simulink model "DutyRelay"  (Simulink 7.0)
settings: Solver=FixedStepDiscrete  StartTime=0.0  StopTime=inf  FixedStep=0.5  RelTol=1e-3
libraries: SuperLogic x3, simulink x1, RT x1
settings Model: Creator=ugur  LastModifiedBy=xx  SimulationMode=accelerator
settings DataIOCC: LimitDataPoints=off  OutputSaveName=yout_CPID
settings OptimizationCC: InlineInvariantSignals=on
settings DebuggingCC: SaveWithParameterizedLinksMsg=none  SignalResolutionControl=TryResolveAllWithWarning  MultiTaskDSMMsg=warning  MultiTaskCondExecSysMsg=none  StrictBusMsg=None
settings RTWCC: IncludeERTFirstTime=on
settings GRTTargetCC: TargetFcnLib=ansi_tfl_tmw.mat

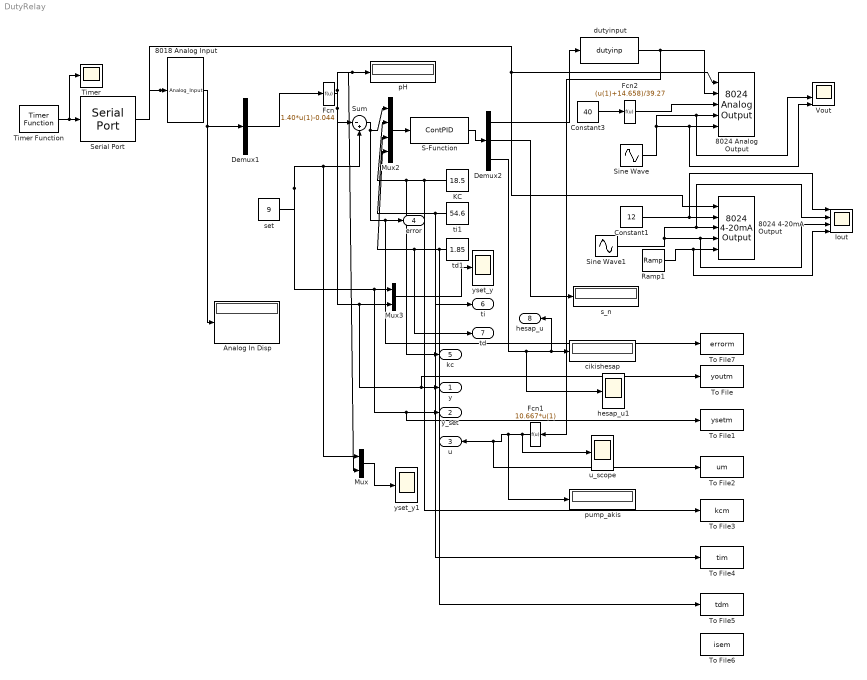
== system DutyRelay ==
  8018 Analog Input : S-Function  FunctionName=Analog_Input  Parameters=AC1, AC2, AC3, AC4, AC5, AC6, AC7, AC8  mask(S function: Analog Input){AC1=off, AC2=on, AC3=off, AC4=off, AC5=off, AC6=off, AC7=off, AC8=off}
      mask prompts: AC1 "Analog Channel 1"; AC2 "Analog Channel 2"; AC3 "Analog Channel 3"; AC4 "Analog Channel 4"; AC5 "Analog Channel 5"; AC6 "Analog Channel 6"; AC7 "Analog Channel 7"; AC8 "Analog Channel 8"
      mask help:
      | This M-file reads the analog input channels from the SL 8018 with 8520
      | The first input is the Com_port number from Serial Port Block.
      mask Display: image(imread('8018.jpg'))
  8024 4-20mA Output : SuperLogic/8024 4-20mA Output  SystemSampleTime=-1  OC1=on  OC2=on  OC3=on  OC4=on
  8024 Analog Output : SuperLogic/8024 Analog Output  SystemSampleTime=-1  OC1=on  OC2=on  OC3=on  OC4=on
  Analog In Disp : Display
  Constant1 : Constant  Value=12  OutDataType=sfix(16)  OutScaling=2^0
  Constant3 : Constant  Value=40  OutDataType=sfix(16)  OutScaling=2^0
  Demux1 : Demux  Outputs=1
  Demux2 : Demux  Outputs=3
  Fcn : Fcn  Expr=1.40*u(1)-0.044
  Fcn1 : Fcn  Orientation=left  Expr=10.667*u(1)
  Fcn2 : Fcn  Expr=(u(1)+14.658)/39.27
  Iout : Scope  NumInputPorts=4
      settings: TimeRange=10  YMin=0~0~0~0  YMax=24~24~24~24  SaveName=ScopeData3  SampleInput=on
  KC : Constant  Orientation=left  Value=18.5  OutDataType=sfix(16)  OutScaling=2^0
  Mux : Mux  Inputs=2
  Mux2 : Mux
  Mux3 : Mux  Inputs=2
  Ramp1 : simulink/Sources/Ramp  SystemSampleTime=-1  slope=0.5  start=0  X0=4
  S-Function : S-Function  FunctionName=ContPID  Parameters=dperiod
  Serial Port : SuperLogic/Serial Port  PORT_NAME=COM1  PORT_BRATE=19200
  Sine Wave : Sin  Amplitude=4  Bias=6  Frequency=pi/5  SampleTime=0
  Sine Wave1 : Sin  Amplitude=8  Bias=12  Frequency=pi/5  SampleTime=0
  Sum : Sum  Inputs=|-+  OutDataType=sfix(16)  OutScaling=2^0
  Timer : Scope
      settings: TimeRange=30  YMin=0  YMax=500
  Timer Function : RT/Timer Function  Priority=245354192  step=500  tmrpriority=HIGH  ThPriority=NORMAL
  To File : ToFile  Filename=youtm
  To File1 : ToFile  Filename=ysetm
  To File2 : ToFile  Filename=um
  To File3 : ToFile  Filename=kcm
  To File4 : ToFile  Filename=tim
  To File5 : ToFile  Filename=tdm
  To File6 : ToFile  Filename=isem
  To File7 : ToFile  Filename=errorm
  Vout : Scope  NumInputPorts=4
      settings: TimeRange=10  YMin=0~0~0~0  YMax=10~10~10~10  SaveName=ScopeData2  SampleInput=on
  cikishesap : Display
  dutyinput : S-Function  FunctionName=dutyinp  Parameters=pumpMax
  hesap_u1 : Scope
      settings: TimeRange=10000  YMin=-60  YMax=70  SaveName=ScopeData6  SampleInput=on
  pH : Display
  pump_akis : Display
  s_n : Display
  set : Constant  Value=9  OutDataType=sfix(16)  OutScaling=2^0
  td1 : Constant  Orientation=left  Value=1.85  OutDataType=sfix(16)  OutScaling=2^0
  ti1 : Constant  Orientation=left  Value=54.6  OutDataType=sfix(16)  OutScaling=2^0
  u_scope : Scope
      settings: TimeRange=10000  YMin=0  YMax=110  SaveName=ScopeData4  SampleInput=on
  yset_y : Scope
      settings: TimeRange=10000  YMin=4.5  YMax=9.5  SampleInput=on
  yset_y1 : Scope
      settings: TimeRange=3000  YMin=0  YMax=300  SaveName=ScopeData5  SampleInput=on
  y : Outport  OutDataType=sfix(16)  OutScaling=2^0
  y_set : Outport  Port=2  OutDataType=sfix(16)  OutScaling=2^0
  u : Outport  Orientation=left  Port=3  OutDataType=sfix(16)  OutScaling=2^0
  error : Outport  Port=4  OutDataType=sfix(16)  OutScaling=2^0
  kc : Outport  Port=5  OutDataType=sfix(16)  OutScaling=2^0
  ti : Outport  Port=6  OutDataType=sfix(16)  OutScaling=2^0
  td : Outport  Port=7  OutDataType=sfix(16)  OutScaling=2^0
  hesap_u : Outport  Orientation=left  Port=8  OutDataType=sfix(16)  OutScaling=2^0
  wires:
  Serial Port/1 -> 8018 Analog Input/1, 8024 4-20mA Output/1, 8024 Analog Output/1
  Timer Function/1 -> Serial Port/1, Timer/1
  8018 Analog Input/1 -> Analog In Disp/1, Demux1/1
  Constant1/1 -> Iout/1, 8024 4-20mA Output/2
  Ramp1/1 -> 8024 4-20mA Output/5, Iout/4
  Sine Wave/1 -> 8024 Analog Output/4, Vout/3, 8024 Analog Output/5, Vout/4
  Sine Wave1/1 -> 8024 4-20mA Output/3, Iout/2, 8024 4-20mA Output/4, Iout/3
  set/1 -> Mux3/1, y_set/1, To File1/1, Mux/1, Sum/2
  Fcn/1 -> Sum/1, pH/1, Mux/2, Mux3/2, y/1, To File/1
  S-Function/1 -> Demux2/1
  Sum/1 -> Mux2/1, error/1, To File7/1
  Mux2/1 -> S-Function/1
  Demux1/1 -> Fcn/1
  Demux2/2 -> s_n/1
  Demux2/3 -> cikishesap/1, hesap_u/1, hesap_u1/1
  Fcn1/1 -> pump_akis/1, u/1, To File2/1, u_scope/1
  Constant3/1 -> Fcn2/1
  Fcn2/1 -> 8024 Analog Output/3
  Mux/1 -> yset_y1/1
  Mux3/1 -> yset_y/1
  KC/1 -> Mux2/2, kc/1, To File3/1
  ti1/1 -> Mux2/3, ti/1, To File4/1
  td1/1 -> Mux2/4, td/1, To File5/1
  Demux2/1 -> dutyinput/1
  dutyinput/1 -> 8024 Analog Output/2, Fcn1/1
